simulink model "A16_PD_Lageregelung"  (R2017b)
settings: Solver=ode45  StartTime=0.0  StopTime=5  MaxStep=1e-4  RelTol=1e-3  EnableMultiTasking=on
model workspace (MAT data in the model file):
  CM = 7.1e-07
  JL = 0.0002
  JR = 1.32e-06
  KM = 0.0384
  KN = 4.15
  LA = 0.000464
  MW = 0.001
  R = 0.02
  RA = 4.99
  Umax = 24
  n0 = 0.01
undefined symbols (not defined in the file or in its folder): sigbuilder_block
libraries: simulink x2
settings Model: Creator=jbaur  LastModifiedBy=jbaur
settings DataIOCC: ExternalInput=X1  SaveFormat=StructureWithTime  InspectSignalLogs=on  SignalLoggingName=sigsOut
settings OptimizationCC: ExpressionDepthLimit=2147483647  InitFltsAndDblsToZero=on  LifeSpan=inf
settings DebuggingCC: SaveWithParameterizedLinksMsg=none  SignalResolutionControl=TryResolveAllWithWarning  MultiTaskDSMMsg=warning  MultiTaskCondExecSysMsg=none  StateNameClashWarn=warning  SFUnexpectedBacktrackingDiag=warning  SFNoUnconditionalDefaultTransitionDiag=warning  SFExecutionAtInitializationDiag=none
settings HardwareCC: ProdBitPerPointer=32  ProdBitPerSizeT=32  ProdBitPerPtrDiffT=32  ProdLargestAtomicFloat=None  ProdIntDivRoundTo=Undefined  ProdEndianess=Unspecified  ProdWordSize=32  ProdHWDeviceType=32-bit Generic  TargetUnknown=on
settings ModelReferenceCC: PropagateSignalLabelsOutOfModel=off
settings CodeAppCC: StateflowObjectComments=on
settings GRTTargetCC: TargetFcnLib=ansi_tfl_tmw.mat  TargetLangStandard=C89/C90 (ANSI)  ModelReferenceCompliant=off  GeneratePreprocessorConditionals=Disable all  CombineOutputUpdateFcns=off  MatFileLogging=off  GRTInterface=on
settings ConfigComp: CovMetricSettings=dw  CovHtmlReporting=on  CovSaveCumulativeToWorkspaceVar=on  CovSaveSingleToWorkspaceVar=on  CovExternalEMLEnable=off  CovSFcnEnable=off

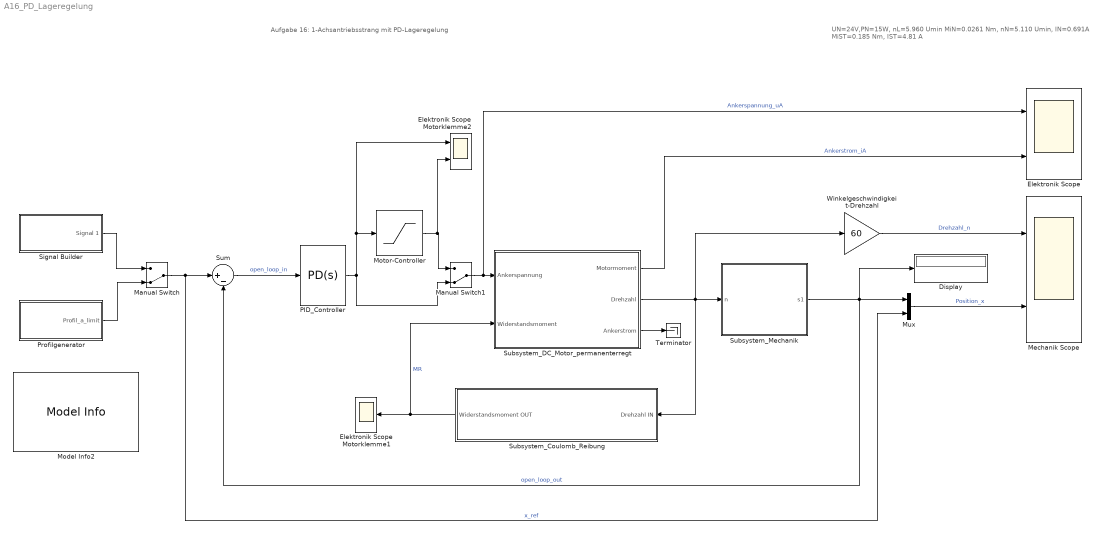
== system A16_PD_Lageregelung ==
  note: Aufgabe 16: 1-Achsantriebsstrang mit PD-Lageregelung
  note: UN=24V,PN=15W, nL=5.960 Umin
      | MiN=0.0261 Nm, nN=5.110 Umin, IN=0.691A
      | MiST=0.185 Nm, IST=4.81 A
  Display : Display
  Elektronik Scope : Scope  NumInputPorts=2
  Elektronik Scope Motorklemme1 : Scope
  Elektronik Scope Motorklemme2 : Scope  NumInputPorts=2
  Manual Switch : ManualSwitch  CurrentSetting=0
  Manual Switch1 : ManualSwitch  CurrentSetting=0
  Mechanik Scope : Scope  NumInputPorts=2
  Model Info2 : simulink/Model-Wide Utilities/Model Info  Frame=on  DisplayStringWithTags=|  HorizontalTextAlignment=Left  LeftAlignmentValue=0.02
      | Bewegungsprofil:
      | ------------------------
      | Tmax = 0.6s
      | smax = 1m
  Motor-Controller : Saturate  UpperLimit=Umax  LowerLimit=-Umax
  Mux : Mux  Inputs=2
  PID_Controller : simulink/Continuous/PID Controller  Controller=PD  TimeDomain=Continuous-time  SampleTime=-1  IntegratorMethod=Forward Euler  FilterMethod=Forward Euler  Form=Ideal  UseFilter=on  ControllerParametersSource=internal  P=8000  I=0  D=0.012  N=190  InitialConditionSource=internal  InitialConditionForIntegrator=0  InitialConditionForFilter=0  ExternalReset=none  LimitOutput=off  UpperSaturationLimit=Umax  LowerSaturationLimit=-Umax  LinearizeAsGain=off  AntiWindupMode=clamping  Kb=1  TrackingMode=off  Kt=1  PParamMin=[]  PParamMax=[]  IParamMin=[]  IParamMax=[]  DParamMin=[]  DParamMax=[]  NParamMin=[]  NParamMax=[]  KbParamMin=[]  KbParamMax=[]  KtParamMin=[]  KtParamMax=[]  POutMin=[]  POutMax=[]  IOutMin=[]  IOutMax=[]  DOutMin=[]  DOutMax=[]  NOutMin=[]  NOutMax=[]  KbOutMin=[]  KbOutMax=[]  KtOutMin=[]  KtOutMax=[]  IntegratorOutMin=[]  IntegratorOutMax=[]  FilterOutMin=[]  FilterOutMax=[]  SumOutMin=[]  SumOutMax=[]  SumI1OutMin=[]  SumI1OutMax=[]  SumI2OutMin=[]  SumI2OutMax=[]  SumI3OutMin=[]  SumI3OutMax=[]  SumDOutMin=[]  SumDOutMax=[]  SaturationOutMin=[]  SaturationOutMax=[]  IntegratorContinuousStateAttributes=''  IntegratorStateMustResolveToSignalObject=off  IntegratorRTWStateStorageClass=Auto  FilterContinuousStateAttributes=''  FilterStateMustResolveToSignalObject=off  FilterRTWStateStorageClass=Auto  DifferentiatorICPrevScaledInput=0  DifferentiatorOutMin=[]  DifferentiatorOutMax=[]  InitialConditionSetting=State (most efficient)  FilterDiffOutCoefMin=[]  FilterDiffOutCoefMax=[]  SumDenOutMin=[]  SumDenOutMax=[]  SumNumOutMin=[]  SumNumOutMax=[]  ReciprocalOutMin=[]  ReciprocalOutMax=[]  DivideOutMin=[]  DivideOutMax=[]  TunerSelectOption=Transfer Function Based (PID Tuner App)
  Profilgenerator : Subsystem
  Signal Builder : Subsystem  Tag=STV Subsys  LoadFcn=sigbuilder_block('load');  StartFcn=sigbuilder_block('start');  StopFcn=sigbuilder_block('stop');  ClipboardFcn=sigbuilder_block('clipboard');  mask(Sigbuilder block){tuvar=[0:10]}
      mask help: Simulink:masks:SigbuilderBlock_MD
      mask init:
      | if ~strcmp(get_param(bdroot(gcbh),'SimulationStatus'),'stopped') tuvar = sigbuilder_block('maskInit'); end
      settings: CopyFcn=sigbuilder_block('copy');  DeleteFcn=sigbuilder_block('delete');  ModelCloseFcn=sigbuilder_block('modelClose');  PreSaveFcn=sigbuilder_block('preSave');  PauseFcn=sigbuilder_block('pause');  ContinueFcn=sigbuilder_block('continue');  NameChangeFcn=sigbuilder_block('namechange');  OpenFcn=sigbuilder_block('open',[437.6 199.2 550.4 400 ]);  CloseFcn=sigbuilder_block('close');
      mask Display: plot(0, 0, 100, 100,[2, 2, 32, 32, 2], [68, 8, 8, 68, 68],[32, 2], [38, 38], [32, 19, 2],[53, 60, 44], [32, 17, 17, 2],[16, 16, 31, 31]);txt = getActiveGroup(gcbh);text(2, 100, txt,'verticalAlignment', 'top');
  Subsystem_Coulomb_Reibung : Subsystem
  Subsystem_DC_Motor_permanenterregt : Subsystem
  Subsystem_Mechanik : Subsystem
  Sum : Sum  Inputs=|+-
  Terminator : Terminator
  Winkelgeschwindigkeit-Drehzahl : Gain  Gain=60
  wires:
  Profilgenerator/1(Profil_a_limit) -> Manual Switch/2
  Signal Builder/1(Signal 1) -> Manual Switch/1
  Manual Switch/1 -> Sum/1, Mux/2  "x_ref"
  Sum/1 -> PID_Controller/1  "open_loop_in"
  Subsystem_Mechanik/1(s1) -> Sum/2, Display/1, Mux/1  "open_loop_out"
  Subsystem_DC_Motor_permanenterregt/2(Drehzahl) -> Winkelgeschwindigkeit-Drehzahl/1, Subsystem_Mechanik/1(n), Subsystem_Coulomb_Reibung/1(Drehzahl IN)
  Subsystem_Coulomb_Reibung/1(Widerstandsmoment OUT) -> Subsystem_DC_Motor_permanenterregt/2(Widerstandsmoment), Elektronik Scope Motorklemme1/1  "MR"
  Mux/1 -> Mechanik Scope/2  "Position_x"
  Subsystem_DC_Motor_permanenterregt/3(Ankerstrom) -> Terminator/1
  Winkelgeschwindigkeit-Drehzahl/1 -> Mechanik Scope/1  "Drehzahl_n"
  Manual Switch1/1 -> Subsystem_DC_Motor_permanenterregt/1(Ankerspannung), Elektronik Scope/1  "Ankerspannung_uA"
  Motor-Controller/1 -> Elektronik Scope Motorklemme2/2, Manual Switch1/1
  PID_Controller/1 -> Manual Switch1/2, Elektronik Scope Motorklemme2/1, Motor-Controller/1
  Subsystem_DC_Motor_permanenterregt/1(Motormoment) -> Elektronik Scope/2  "Ankerstrom_iA"

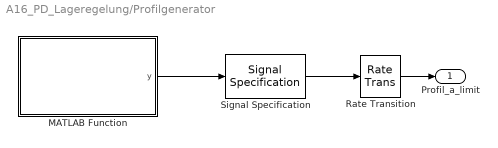
== system A16_PD_Lageregelung/Profilgenerator ==
  MATLAB Function : MATLAB Function  TreatAsAtomicUnit=on
  Rate Transition : RateTransition
  Signal Specification : SignalSpecification  SampleTime=1e-4
  Profil_a_limit : Outport
  wires:
  Signal Specification/1 -> Rate Transition/1
  MATLAB Function/1(y) -> Signal Specification/1
  Rate Transition/1 -> Profil_a_limit/1

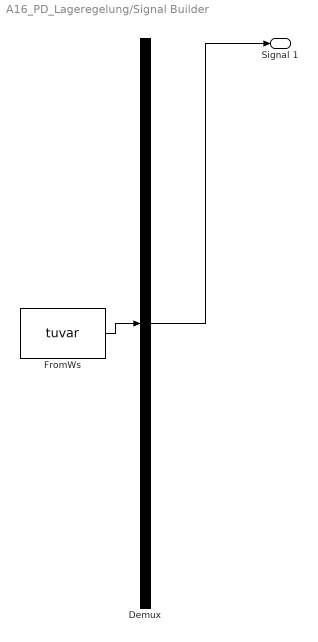
== system A16_PD_Lageregelung/Signal Builder ==
  Demux : Demux  Tag=STV Demux  Outputs=1
  FromWs : FromWorkspace  Tag=STV FromWs  VariableName=tuvar  SampleTime=0
      SigBuilderData=|
      | common.afterFinalStr = 'Extrapolate'
      | common.sampleTime = 0
      | dataSet.timeRange = [0 10]
      | dataSet.name = 'Group 1'
      | sbobj.Groups.Name = 'Group 1'
      | sbobj.Groups.Signals.Name = 'Signal 1'
      | sbobj.Groups.Signals.XData = [0 1 1 2 3 10]
      | sbobj.Groups.Signals.YData = [0 0 1 1 0 0]
  Signal 1 : Outport  Tag=STV Outport
  wires:
  Demux/1 -> Signal 1/1
  FromWs/1 -> Demux/1

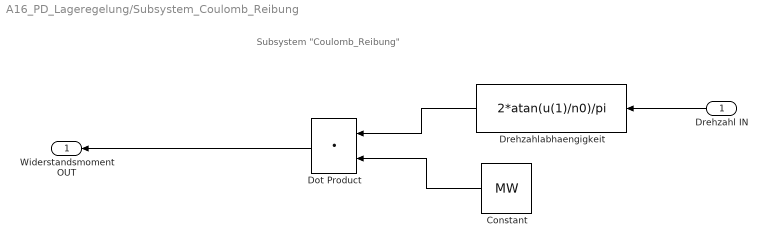
== system A16_PD_Lageregelung/Subsystem_Coulomb_Reibung ==
  note: Subsystem "Coulomb_Reibung"
  Drehzahl IN : Inport
  Constant : Constant  Value=MW
  Dot Product : DotProduct  InputSameDT=on  OutDataTypeStr=Inherit: Inherit via internal rule
  Drehzahlabhaengigkeit : Fcn  Expr=2*atan(u(1)/n0)/pi
  Widerstandsmoment OUT : Outport
  wires:
  Drehzahl IN/1 -> Drehzahlabhaengigkeit/1
  Drehzahlabhaengigkeit/1 -> Dot Product/1
  Constant/1 -> Dot Product/2
  Dot Product/1 -> Widerstandsmoment OUT/1

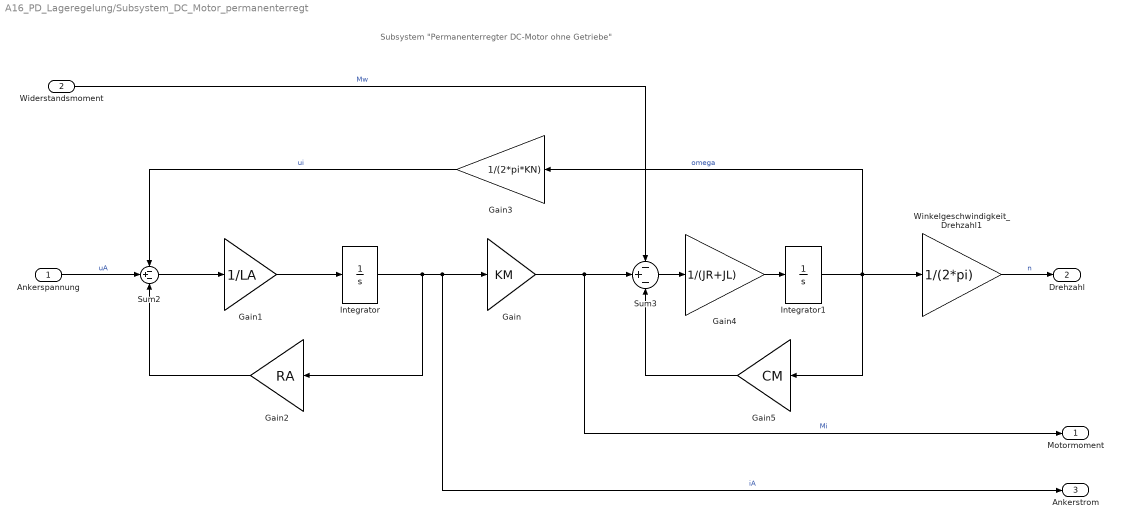
== system A16_PD_Lageregelung/Subsystem_DC_Motor_permanenterregt ==
  note: Subsystem "Permanenterregter DC-Motor ohne Getriebe"
  Ankerspannung : Inport
  Widerstandsmoment : Inport  Port=2
  Gain : Gain  Gain=KM
  Gain1 : Gain  Gain=1/LA
  Gain2 : Gain  Gain=RA
  Gain3 : Gain  Gain=1/(2*pi*KN)
  Gain4 : Gain  Gain=1/(JR+JL)
  Gain5 : Gain  Gain=CM
  Integrator : Integrator
  Integrator1 : Integrator
  Sum2 : Sum  Inputs=-+-
  Sum3 : Sum  Inputs=-+-
  Winkelgeschwindigkeit_Drehzahl1 : Gain  Gain=1/(2*pi)
  Motormoment : Outport
  Drehzahl : Outport  Port=2
  Ankerstrom : Outport  Port=3
  wires:
  Ankerspannung/1 -> Sum2/2  "uA"
  Gain3/1 -> Sum2/1  "ui"
  Gain/1 -> Sum3/2, Motormoment/1  "Mi"
  Winkelgeschwindigkeit_Drehzahl1/1 -> Drehzahl/1  "n"
  Sum2/1 -> Gain1/1
  Gain1/1 -> Integrator/1
  Integrator/1 -> Gain2/1, Ankerstrom/1, Gain/1  "iA"
  Sum3/1 -> Gain4/1
  Gain4/1 -> Integrator1/1
  Integrator1/1 -> Gain3/1, Winkelgeschwindigkeit_Drehzahl1/1, Gain5/1  "omega"
  Gain5/1 -> Sum3/3
  Gain2/1 -> Sum2/3
  Widerstandsmoment/1 -> Sum3/1  "Mw"

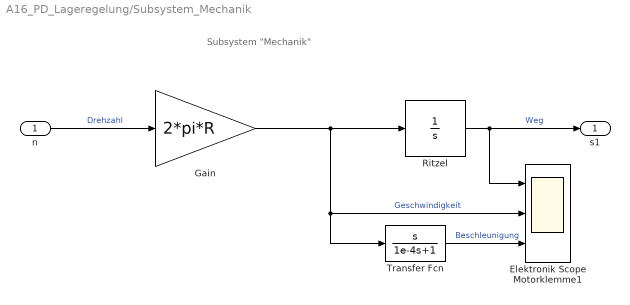
== system A16_PD_Lageregelung/Subsystem_Mechanik ==
  note: Subsystem "Mechanik"
  n : Inport
  Elektronik Scope Motorklemme1 : Scope  NumInputPorts=3
  Gain : Gain  Gain=2*pi*R
  Ritzel : TransferFcn  Denominator=[1 0]
  Transfer Fcn : TransferFcn  Numerator=[1 0]  Denominator=[1e-4 1]
  s1 : Outport
  wires:
  Ritzel/1 -> Elektronik Scope Motorklemme1/1, s1/1  "Weg"
  n/1 -> Gain/1  "Drehzahl"
  Gain/1 -> Transfer Fcn/1, Elektronik Scope Motorklemme1/2, Ritzel/1  "Geschwindigkeit"
  Transfer Fcn/1 -> Elektronik Scope Motorklemme1/3  "Beschleunigung"

== matlab function A16_PD_Lageregelung/Profilgenerator/MATLAB Function ==
  data: y output
function y = Zeitfunktion
% This block supports an embeddable subset of the MATLAB language.
% See the help menu for details. 

% Deklaration der persistenten (globalen) Zeitvariablen
Timestep = 1e-4;
persistent t

% Definition der Zeitfunktion
if isempty(t)
    t=0;
  else
    t = t + Timestep;
end

% Dreiecksprofil fuer Geschwindigkeit
% (keine gleichförmige Bewegung)
s_max = 1;
T_max = 0.6;
t1 = T_max/2;
a_max = s_max/t1^2;
v_max = a_max*t1;

% Bereichsunterscheidung
if t<=t1
    y = 0.5*a_max*t^2;
else
    if t <= T_max
        y = 0.5*s_max + v_max*(t-t1) - 0.5*a_max*(t-t1)^2;
    else
        y = s_max;
    end
end
